simulink model "Simple_TDMA_test"  (Simulink 9.0)
settings: Solver=VariableStepAuto  StartTime=0.0  StopTime=1.0000e-04  RelTol=1e-3  EnableMultiTasking=on
undefined symbols (not defined in the file or in its folder): paramRFSatLink
libraries: commrflib2 x6, dspsigops x3, commrfcorlib x2, commrandsrc3 x2, dspsolvers x2, simulink x2, commfilt2 x2, commdigbbndam3 x2, commsink2 x1, commsync2 x1, commblksprivate x1
settings Model: SuppressorTable=22 serialization::archive 11 0 6 0 0 0 0 0  Creator=15337  LastModifiedBy=changgang
settings DataIOCC: LimitDataPoints=on  SaveFormat=Dataset
settings DebuggingCC: UnderspecifiedInitializationDetection=Simplified  MergeDetectMultiDrivingBlocksExec=error  AllowSymbolicDim=off
settings HardwareCC: ProdBitPerPointer=64  ProdBitPerSizeT=64  ProdBitPerPtrDiffT=64  ProdLargestAtomicFloat=Float  ProdIntDivRoundTo=Zero  ProdEndianess=LittleEndian  ProdWordSize=64  ProdHWDeviceType=Intel->x86-64 (Windows64)

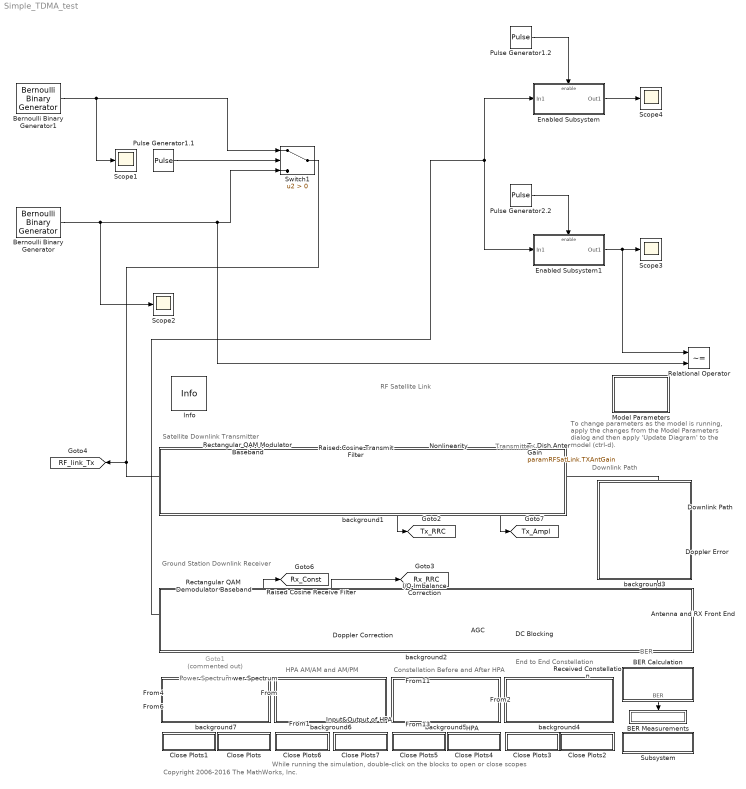
== system Simple_TDMA_test ==
  note: HPA AM/AM and AM/PM
  note: While running the simulation, double-click on the blocks to open or close scopes
  note: BER
  note: Power Spectrum
  note: Downlink Path
  note: RF Satellite Link
  note: Constellation Before and
      | After HPA
  note: End to End Constellation
  note: Ground Station Downlink Receiver
  note: Transmitter
  note: Satellite Downlink Transmitter
  note: Copyright 2006-2016 The MathWorks, Inc.
  note: To change parameters as the model is running, apply the changes from the Model Parameters dialog and then apply 'Update Diagram' to the model (ctrl-d).
  AGC : commrfcorlib/AGC  LegacyMode=off  DetectorMethod=Rectifier  LoopMethod=Linear  UpdatePeriod=100  StepSize=0.1  AdaptationStepSize=0.01  DesiredOutputPower=1  AveragingLength=256  MaximumGain=30  MaxPowerGain=400  GainOutputPort=off  InputPowerOutputPort=off  SimulateUsing=Code generation
      settings: SourceProductName=Communications System Toolbox
  Antenna and RX Front End : Subsystem
      mask Display: disp('Antenna and\nRX Front End')
  BER Calculation : Subsystem
      mask Display: disp('Display Complete\nBit Error Rate\nInformation');
  BER Measurements : Display
      settings: Format=short_e
  Bernoulli Binary Generator : commrandsrc3/Bernoulli Binary Generator  ProbabilityOfZero=0.5  SeedSource=Parameter  Seed=37  SampleTime=paramRFSatLink.sourceSampleTime  SamplesPerFrame=paramRFSatLink.sourceSamplesPerSymbol  OutputDataType=double  SimulateUsing=Interpreted execution
  Bernoulli Binary Generator1 : commrandsrc3/Bernoulli Binary Generator  ProbabilityOfZero=0.5  SeedSource=Parameter  Seed=37  SampleTime=paramRFSatLink.sourceSampleTime  SamplesPerFrame=paramRFSatLink.sourceSamplesPerSymbol  OutputDataType=double  SimulateUsing=Interpreted execution
  Close Plots : Subsystem
      settings: OpenFcn=|
      | sdspfscope2([],[],[],'ScopeUpdate',[bdroot '/Power Spectrum/Tx and Rx Spectrum'],'CloseFig');
      | set_param([bdroot '/Power Spectrum/Tx and Rx Spectrum'],'OpenScopeAtSimStart','off');
      mask Display: disp('Close Scopes');
  Close Plots1 : Subsystem
      settings: OpenFcn=|
      | sdspfscope2([],[],[],'ScopeUpdate',[bdroot '/Power Spectrum/Tx and Rx Spectrum'],'OpenFig');
      | set_param([bdroot '/Power Spectrum/Tx and Rx Spectrum'],'OpenScopeAtSimStart','on');
      mask Display: disp('Open Scopes');
  Close Plots2 : Subsystem
      settings: OpenFcn=|
      | sdspfscope2([],[],[],'ScopeUpdate',[bdroot '/Received Constellation'],'CloseFig');
      |    set_param([bdroot '/Received Constellation'],'OpenScopeAtSimStart','off');
      mask Display: disp('Close Scopes');
  Close Plots3 : Subsystem
      settings: OpenFcn=|
      | sdspfscope2([],[],[],'ScopeUpdate',[bdroot '/Received Constellation'],'OpenFig');
      |     set_param([bdroot '/Received Constellation'],'OpenScopeAtSimStart','on');
      mask Display: disp('Open Scopes');
  Close Plots4 : Subsystem
      settings: OpenFcn=|
      | sdspfscope2([],[],[],'ScopeUpdate',[bdroot '/HPA/Transmit RRC filtered signal'],'CloseFig');
      |   set_param([bdroot '/HPA/Transmit RRC filtered signal'],'OpenScopeAtSimStart','off');
      |     sdspfscope2([],[],[],'ScopeUpdate',[bdroot '/HPA/RRC signal after HPA'],'CloseFig');
      |   set_param([bdroot '/HPA/RRC signal after HPA'],'OpenScopeAtSimStart','off');
      mask Display: disp('Close Scopes');
  Close Plots5 : Subsystem
      settings: OpenFcn=|
      | sdspfscope2([],[],[],'ScopeUpdate',[bdroot '/HPA/Transmit RRC filtered signal'],'OpenFig');
      | set_param([bdroot '/HPA/Transmit RRC filtered signal'],'OpenScopeAtSimStart','on');
      |   sdspfscope2([],[],[],'ScopeUpdate',[bdroot '/HPA/RRC signal after HPA'],'OpenFig');
      | set_param([bdroot '/HPA/RRC signal after HPA'],'OpenScopeAtSimStart','on');
      mask Display: disp('Open Scopes');
  Close Plots6 : Subsystem
      settings: OpenFcn=|
      | sdspfscope2([],[],[],'ScopeUpdate',[bdroot '/Input&Output of HPA/HPA AM to AM'],'OpenFig');
      | set_param([bdroot '/Input&Output of HPA/HPA AM to AM'],'OpenScopeAtSimStart','on');
      | sdspfscope2([],[],[],'ScopeUpdate',[bdroot '/Input&Output of HPA/HPA AM to PM'],'OpenFig');
      | set_param([bdroot '/Input&Output of HPA/HPA AM to PM'],'OpenScopeAtSimStart','on');
      mask Display: disp('Open Scopes');
  Close Plots7 : Subsystem
      settings: OpenFcn=|
      | sdspfscope2([],[],[],'ScopeUpdate',[bdroot '/Input&Output of HPA/HPA AM to AM'],'CloseFig');
      | set_param([bdroot '/Input&Output of HPA/HPA AM to AM'],'OpenScopeAtSimStart','off');
      | sdspfscope2([],[],[],'ScopeUpdate',[bdroot '/Input&Output of HPA/HPA AM to PM'],'CloseFig');
      | set_param([bdroot '/Input&Output of HPA/HPA AM to PM'],'OpenScopeAtSimStart','off');
      mask Display: disp('Close Scopes');
  DC Blocking : Subsystem
      mask Display: disp('DC Blocking')
  Doppler Correction : Subsystem
      mask Display: disp('Doppler\nCorrection')
  Doppler Error : commrflib2/Phase// Frequency Offset  phaseOffset=0  freqPort=off  freqOffset=paramRFSatLink.DoppOffset
      settings: SourceProductName=Communications System Toolbox
  Downlink Path : commrflib2/Free Space Path Loss  mode=Distance and Frequency  dB=180  d=paramRFSatLink.Altitude  fc=paramRFSatLink.Frequency
      settings: SourceProductName=Communications System Toolbox  SourceProductBaseCode=CM
  Enabled Subsystem : Subsystem  TreatAsAtomicUnit=on
  Enabled Subsystem1 : Subsystem  TreatAsAtomicUnit=on
  Goto1 : Goto  Commented=on  GotoTag=RF_link_Rx  TagVisibility=global
  HPA : Subsystem  TreatAsAtomicUnit=on
      mask Display: disp('HPA\nConstellation')
  I/Q Imbalance Correction : Subsystem
      mask Display: disp('I/Q Imbalance\nCorrection')
  Info : commblksprivate/Info  SystemSampleTime=-1
      settings: SourceProductName=Communications System Toolbox  SourceProductBaseCode=CM
  Input&Output of HPA : Subsystem
      mask Display: disp('Input/Output\nof HPA')
  Model Parameters : Subsystem  mask(Model Parameters){altitude=35600, frequency=4000, antDiam=[.4 .4], selTemp=20 (very low noise level), selLvlBO=30 dB  (negligible nonlinearity), selDoppler=0 Hz, selNoPh=Negligible (-100 dBc/Hz @ 100 Hz), selImbal=None, selPreDistortion=off, selDcOffset=off, selCorrIQ=off, selCorrDoppler=off}
      mask prompts: altitude "Satellite altitude (km):"; frequency "Frequency (MHz):"; antDiam "Transmit and receive antenna diameters (m):"; selTemp "Noise temperature (K):"; selLvlBO "HPA backoff level:"; selDoppler "Doppler error:"; selNoPh "Phase noise:"; selImbal "I/Q imbalance and DC offset:"; selPreDistortion "Digital predistortion"; selDcOffset "DC offset correction"; selCorrIQ "I/Q imbalance correction"; selCorrDoppler "Doppler correction"
      mask help:
      | Select the scenarios from the mask to change the link parameters. Each of the mask parameters sets the parameters in the corresponding RF impairment or corresponding correction block(s).
      |
      | To make changes as the model is running, apply the changes from this dialog and then apply Update Diagram to the model (crtl-d).
      mask init:
      | commrfsatlink_mask(selLvlBO,selTemp, ...
      |     selDoppler, selImbal, selNoPh, ...
      |     selDcOffset, selCorrDoppler, selCorrIQ, altitude, ...
      |     frequency, antDiam,8,6,selPreDistortion);
      mask Help: helpview(commdhelp);
      mask TypeOptions selTemp: 0 (no noise) | 20 (very low noise level) | 290 (typical noise level) | 500 (high noise level)
      mask TypeOptions selLvlBO: 30 dB  (negligible nonlinearity) | 7 dB  (moderate nonlinearity) | 1 dB  (severe nonlinearity)
      mask TypeOptions selDoppler: 0 Hz | 3 Hz
      mask TypeOptions selNoPh: Negligible (-100 dBc/Hz @ 100 Hz) | Low  (-55 dBc/Hz @ 100 Hz) | High  (-48 dBc/Hz @ 100 Hz)
      mask TypeOptions selImbal: None | Amplitude imbalance (3 dB) | Phase imbalance (20 deg) | In-phase DC offset (2e-6) | Quadrature DC offset (1e-5)
      mask Display: disp('Model\nParameters');
  Nonlinearity : Subsystem
      mask Display: disp('HPA\n Nonlinearity\n with Optional\n Digital\nPredistortion')
  Power Spectrum : Subsystem  TreatAsAtomicUnit=on
      mask Display: disp('Power\nSpectrum')
  Pulse Generator1.1 : DiscretePulseGenerator  PulseType=Time based  Period=5.0000e-06  PulseWidth=50
  "Pulse Generator1.2 " : DiscretePulseGenerator  PulseType=Time based  Period=1.0000e-05  PulseWidth=50
  Pulse Generator2.2 : DiscretePulseGenerator  PulseType=Time based  Period=1.0000e-05  PulseWidth=50  PhaseDelay=0.05
  Raised Cosine Receive Filter : commfilt2/Raised Cosine Receive Filter  filtType=Square root  R=0.3  filtSpan=paramRFSatLink.FilterSpan  N=paramRFSatLink.SamplesPerSymbol  downFactor=paramRFSatLink.SamplesPerSymbol  downOffset=0  filterGain=1/sqrt(paramRFSatLink.SamplesPerSymbol)  InputProcessing=Columns as channels (frame based)  RateOptions=Enforce single-rate processing  framing=Mute  checkCoeff=off  variableName=rcRxFilt  currentFiltSpan=2*((2*(3))/2)  D=(2*(3))/2  inputOffset=0  sampMode=Mute  saveAsFlag=0  rateMode=Downsampling  checkGain=Normalized  launchFVT=off  roundingMode=Floor  overflowMode=off  coeffDataTypeStr=Inherit: Same word length as input  coeffMin=[]  coeffMax=[]  coeffLastDataTypeStr=Inherit: Same word length as input  accumDataTypeStr=Inherit: Same as product output  accumLastDataTypeStr=Inherit: Same as product output  outputDataTypeStr=Inherit: Same as accumulator  outputMin=[]  outputMax=[]  outputLastDataTypeStr=Inherit: Same as accumulator
  Raised Cosine Transmit Filter : commfilt2/Raised Cosine Transmit Filter  filtType=Square root  R=0.3  filtSpan=paramRFSatLink.FilterSpan  N=paramRFSatLink.SamplesPerSymbol  filterGain=sqrt(paramRFSatLink.SamplesPerSymbol)  InputProcessing=Columns as channels (frame based)  RateOptions=Enforce single-rate processing  framing=Mute  checkCoeff=off  variableName=rcTxFilt  checkGain=Normalized  sampMode=Mute  saveAsFlag=0  currentFiltSpan=2*((2*(3))/2)  D=(2*(3))/2  launchFVT=off  roundingMode=Floor  overflowMode=off  coeffDataTypeStr=Inherit: Same word length as input  coeffMin=[]  coeffMax=[]  coeffLastDataTypeStr=Inherit: Same word length as input  outputDataTypeStr=Inherit: Same as accumulator  outputMin=[]  outputMax=[]  outputLastDataTypeStr=Inherit: Same as accumulator
  Received Constellation : ConstellationDiagram  Tag=ScatterPlot
  Rectangular QAM Demodulator Baseband : commdigbbndam3/Rectangular QAM Demodulator Baseband  M=16  OutType=Bit  DecType=Hard decision  VarSource=Dialog  Variance=1  Dec=Gray  Mapping=[0:15]  PowType=Average Power  MinDist=2  AvgPow=1  PeakPow=1  Ph=0  outDtype1=boolean  outDtype2=double  derotateFactorWordLen=16  derotateFactorDataTypeStr=Inherit: Same word length as input  derotateFactorLastDataTypeStr=Inherit: Same word length as input  denormFactorWordLen=16  denormFactorDataTypeStr=Inherit: Same word length as input  denormFactorLastDataTypeStr=Inherit: Same word length as input  prodOutWordLen=32  prodOutOverflowMode=Wrap  prodOutRoundingMode=Floor  prodOutOvFlMode=off  prodOutOvFlModeLastStrValue=off  sumWordLen=32
  Rectangular QAM Modulator Baseband : commdigbbndam3/Rectangular QAM Modulator Baseband  M=16  InType=Bit  Enc=Gray  Mapping=[0:15]  PowType=Average Power  MinDist=2  AvgPow=1  PeakPow=1  Ph=0  outDtype=double  outWordLen=16  outUDDataType=sfix(16)  outFracLenMode=Best precision  outFracLen=15  outDataTypeStr=double  outLastDataTypeStr=double
  Relational Operator : RelationalOperator  Operator=~=  OutDataTypeStr=boolean  RndMeth=Nearest
  Scope{1..4} (4 alike) : Scope
  Subsystem : Subsystem
      settings: OpenFcn=|
      | % Set value to reset BER
      | warning('off', 'Simulink:Engine:NonTunableVarChanged');
      | paramRFSatLink.resetBER = 1;
      | set_param(bdroot, 'SimulationCommand', 'update');
      | pause(0.1)
      | 
      | % Set value so that BER is not continually reset
      | paramRFSatLink.resetBER = 0;
      | set_param(bdroot, 'SimulationCommand', 'update');
      | warning('on', 'Simulink:Engine:NonTunableVarChanged');
      mask Display: disp('Double-click to\nreset BER')
  Switch1 : Switch  Criteria=u2 > Threshold
  Tx Dish Antenna Gain : Gain  Gain=paramRFSatLink.TXAntGain  SaturateOnIntegerOverflow=on  OutDataTypeStr=Inherit: Same as input  ParamDataTypeStr=Inherit: Same as input
  background1 : Subsystem
      mask Display: disp('')
  background2 : Subsystem
      mask Display: disp('')
  background3 : Subsystem
      mask Display: disp('')
  background4 : Subsystem
      mask Display: disp('')
  background5 : Subsystem
      mask Display: disp('')
  background6 : Subsystem
      mask Display: disp('')
  background7 : Subsystem
      mask Display: disp('')
  tag scope: RF_link_Tx=global, Rx_Const=global, Rx_RRC=global, Tx_Ampl=global, Tx_RRC=global
  wires:
  Pulse Generator1.1/1 -> Switch1/2
  "Pulse Generator1.2 "/1 -> Enabled Subsystem/Enable
  Pulse Generator2.2/1 -> Enabled Subsystem1/Enable
  Bernoulli Binary Generator/1 -> Relational Operator/2, Switch1/3, Scope2/1
  Rectangular QAM Demodulator Baseband/1 -> Enabled Subsystem1/1(In1), Enabled Subsystem/1(In1), Goto1/1
  Enabled Subsystem/1(Out1) -> Scope4/1
  Enabled Subsystem1/1(Out1) -> Relational Operator/1, Scope3/1
  Antenna and RX Front End/1(Out1) -> DC Blocking/1(In1)
  [Tx_Ampl] -> HPA/2(In3)
  BER Calculation/1(BER) -> BER Measurements/1
  [HPA_Out] -> Input&Output of HPA/2(In2)
  [Rx_Const] -> Received Constellation/1
  Doppler Correction/1(Out1) -> [Rx_RRC], Raised Cosine Receive Filter/1
  Downlink Path/1 -> Doppler Error/1
  Raised Cosine Receive Filter/1 -> [Rx_Const], Rectangular QAM Demodulator Baseband/1
  Tx Dish Antenna Gain/1 -> Downlink Path/1
  Doppler Error/1 -> Antenna and RX Front End/1(In1)
  DC Blocking/1(Out1) -> AGC/1
  Switch1/1 -> Rectangular QAM Modulator Baseband/1, [RF_link_Tx]
  [Tx_RRC] -> HPA/1(In2)
  I/Q Imbalance Correction/1(Out1) -> Doppler Correction/1(In1)
  AGC/1 -> I/Q Imbalance Correction/1(In1)
  [HPA_In] -> Input&Output of HPA/1(In1)
  [Rx_RRC] -> Power Spectrum/2(In2)
  Nonlinearity/1(Out2) -> [Tx_Ampl], Tx Dish Antenna Gain/1
  [Tx_RRC] -> Power Spectrum/1(In1)
  Raised Cosine Transmit Filter/1 -> [Tx_RRC], Nonlinearity/1(In)
  Bernoulli Binary Generator1/1 -> Switch1/1, Scope1/1
  Rectangular QAM Modulator Baseband/1 -> Raised Cosine Transmit Filter/1

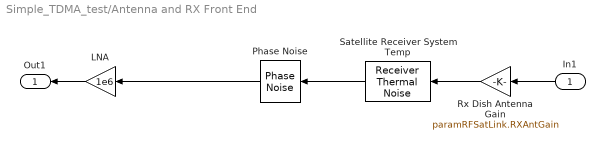
== system Simple_TDMA_test/Antenna and RX Front End ==
  In1 : Inport
  LNA : Gain  Gain=1e6
  Phase Noise : commrflib2/Phase Noise  PhNs=paramRFSatLink.PhaseNoise  Fo=100  Fs=2e5  seed=2137
      settings: SourceProductName=Communications System Toolbox  SourceProductBaseCode=CM
  Rx Dish Antenna Gain : Gain  Gain=paramRFSatLink.RXAntGain  SaturateOnIntegerOverflow=on  OutDataTypeStr=Inherit: Same as input  ParamDataTypeStr=Inherit: Same as input
  Satellite Receiver System Temp : commrflib2/Receiver Thermal Noise  method=Noise temperature  ntemp=paramRFSatLink.RXTemp  nfigure=20  nfactor=2  add290KAntennaNoise=off  seed=67987
      settings: SourceProductName=Communications System Toolbox  SourceProductBaseCode=CM
  Out1 : Outport
  wires:
  LNA/1 -> Out1/1
  Satellite Receiver System Temp/1 -> Phase Noise/1
  In1/1 -> Rx Dish Antenna Gain/1
  Phase Noise/1 -> LNA/1
  Rx Dish Antenna Gain/1 -> Satellite Receiver System Temp/1

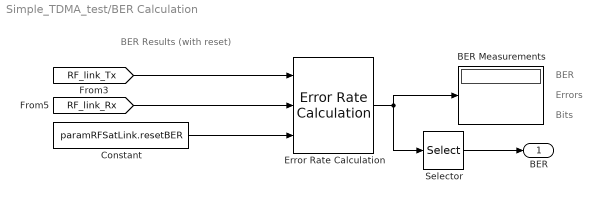
== system Simple_TDMA_test/BER Calculation ==
  note: BER
  note: Errors
  note: Bits
  note: BER Results (with reset)
  BER Measurements : Display
  Constant : Constant  Value=paramRFSatLink.resetBER  SampleTime=paramRFSatLink.sourceSampleTime * paramRFSatLink.sourceSamplesPerSymbol
  Error Rate Calculation : commsink2/Error Rate Calculation  N=24  st_delay=0  cp_mode=Entire frame  subframe=[]  PMode=Port  WsName=ErrorVec  RsMode2=on  stop=off  numErr=200  maxBits=1e6
  Selector : Selector  InputPortWidth=3  IndexOptions=Index vector (dialog)  Indices=[1]  OutputSizes=1
  BER : Outport
  wires:
  [RF_link_Rx] -> Error Rate Calculation/2
  Error Rate Calculation/1 -> Selector/1, BER Measurements/1
  Constant/1 -> Error Rate Calculation/3
  Selector/1 -> BER/1
  [RF_link_Tx] -> Error Rate Calculation/1

== system Simple_TDMA_test/Close Plots ==

== system Simple_TDMA_test/Close Plots1 ==

== system Simple_TDMA_test/Close Plots2 ==

== system Simple_TDMA_test/Close Plots3 ==

== system Simple_TDMA_test/Close Plots4 ==

== system Simple_TDMA_test/Close Plots5 ==

== system Simple_TDMA_test/Close Plots6 ==

== system Simple_TDMA_test/Close Plots7 ==

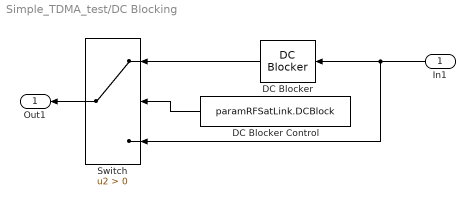
== system Simple_TDMA_test/DC Blocking ==
  In1 : Inport
  DC Blocker : dspsigops/DC Blocker  Algorithm=IIR  NormalizedBandwidth=0.0005  Length=8  Order=6  SimulateUsing=Code generation
      settings: SourceProductName=DSP System Toolbox  SourceProductBaseCode=DS
  DC Blocker Control : Constant  Value=paramRFSatLink.DCBlock  SampleTime=paramRFSatLink.sourceSampleTime * paramRFSatLink.sourceSamplesPerSymbol
  Switch : Switch  Criteria=u2 > Threshold
  Out1 : Outport
  wires:
  In1/1 -> Switch/3, DC Blocker/1
  DC Blocker Control/1 -> Switch/2
  Switch/1 -> Out1/1
  DC Blocker/1 -> Switch/1

== system Simple_TDMA_test/Doppler Correction ==
  In1 : Inport
  Carrier Synchronizer : commsync2/Carrier Synchronizer  Modulation=QAM  ModulationPhaseOffset=Auto  CustomPhaseOffset=0  SamplesPerSymbol=paramRFSatLink.SamplesPerSymbol  DampingFactor=0.707  NormalizedLoopBandwidth=0.01  EstimatedPhaseErrorOutputPort=off  SimulateUsing=Code generation
      settings: SourceProductName=Communications System Toolbox
  Doppler Correction : Constant  Value=paramRFSatLink.CarrierSync  SampleTime=paramRFSatLink.sourceSampleTime * paramRFSatLink.sourceSamplesPerSymbol
  Switch : Switch  Criteria=u2 > Threshold
  Out1 : Outport
  wires:
  Doppler Correction/1 -> Switch/2
  Carrier Synchronizer/1 -> Switch/1
  Switch/1 -> Out1/1
  In1/1 -> Carrier Synchronizer/1, Switch/3

== system Simple_TDMA_test/Enabled Subsystem ==
  In1 : Inport
  Enable : EnablePort
  Out1 : Outport
  wires:
  In1/1 -> Out1/1

== system Simple_TDMA_test/Enabled Subsystem1 ==
  In1 : Inport
  Enable : EnablePort
  Out1 : Outport
  wires:
  In1/1 -> Out1/1

== system Simple_TDMA_test/HPA ==
  In2 : Inport
  In3 : Inport  Port=2
  RRC signal after HPA : ConstellationDiagram
  Transmit RRC filtered signal : ConstellationDiagram
  wires:
  In2/1 -> Transmit RRC filtered signal/1
  In3/1 -> RRC signal after HPA/1

== system Simple_TDMA_test/I/Q Imbalance Correction ==
  In1 : Inport
  I/Q Imbalance Compensator : commrfcorlib/I//Q Imbalance Compensator  CoefficientSource=Estimated from input signal  InitialCoefficient=0 + 0j  StepSizeSource=Property  StepSize=0.00001  AdaptInputPort=off  CoefficientOutputPort=off  SimulateUsing=Code generation
      settings: SourceProductName=Communications System Toolbox  SourceProductBaseCode=CM
  I/Q Imbalance Correction : Constant  Value=paramRFSatLink.IQComp  SampleTime=paramRFSatLink.sourceSampleTime * paramRFSatLink.sourceSamplesPerSymbol
  Switch : Switch  Criteria=u2 > Threshold
  Out1 : Outport
  wires:
  I/Q Imbalance Correction/1 -> Switch/2
  I/Q Imbalance Compensator/1 -> Switch/1
  Switch/1 -> Out1/1
  In1/1 -> I/Q Imbalance Compensator/1, Switch/3

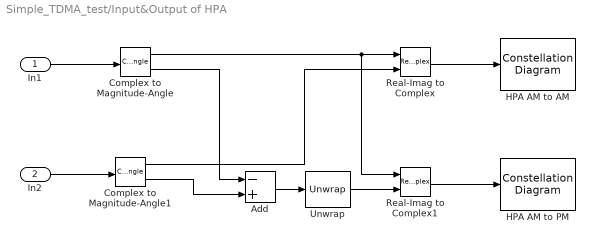
== system Simple_TDMA_test/Input&Output of HPA ==
  In1 : Inport
  In2 : Inport  Port=2
  Add : Sum  Inputs=-+
  Complex to Magnitude-Angle : ComplexToMagnitudeAngle
  Complex to Magnitude-Angle1 : ComplexToMagnitudeAngle
  HPA AM to AM : ConstellationDiagram  Tag=ScatterPlot
  HPA AM to PM : ConstellationDiagram  Tag=ScatterPlot
  Real-Imag to Complex : RealImagToComplex
  Real-Imag to Complex1 : RealImagToComplex
  Unwrap : dspsigops/Unwrap  tol=pi  InputProcessing=Columns as channels (frame based)  running=on
  wires:
  Real-Imag to Complex/1 -> HPA AM to AM/1
  Complex to Magnitude-Angle1/1 -> Real-Imag to Complex/2
  Add/1 -> Unwrap/1
  In1/1 -> Complex to Magnitude-Angle/1
  In2/1 -> Complex to Magnitude-Angle1/1
  Real-Imag to Complex1/1 -> HPA AM to PM/1
  Unwrap/1 -> Real-Imag to Complex1/2
  Complex to Magnitude-Angle1/2 -> Add/2
  Complex to Magnitude-Angle/1 -> Real-Imag to Complex1/1, Real-Imag to Complex/1
  Complex to Magnitude-Angle/2 -> Add/1

== system Simple_TDMA_test/Model Parameters ==

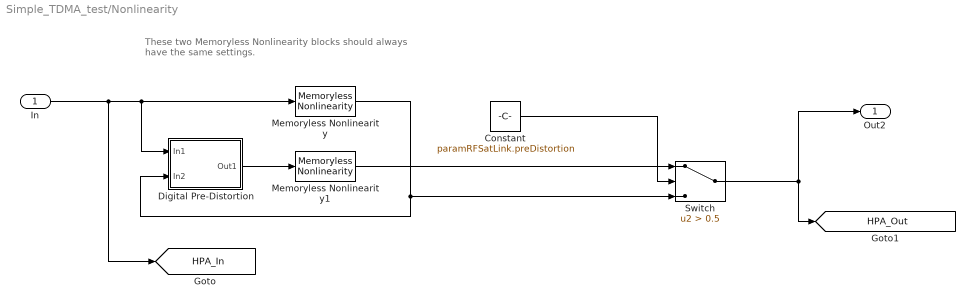
== system Simple_TDMA_test/Nonlinearity ==
  note: These two Memoryless Nonlinearity blocks should always
      | have the same settings.
  In : Inport
  Constant : Constant  Value=paramRFSatLink.preDistortion  VectorParams1D=off  SampleTime=paramRFSatLink.sourceSampleTime * paramRFSatLink.sourceSamplesPerSymbol
  Digital Pre-Distortion : Subsystem
      mask Display: disp('Digital\nPredistortion')
  Memoryless Nonlinearity : commrflib2/Memoryless Nonlinearity  model_select=Saleh model  linGaindB=0  GindB=paramRFSatLink.GindB  iip3=30  am2pm=10  LPwrLimAMPM=10  UPwrLimAMPM=inf  amam=[2.1587 1.1517]  ampm=[4.0330 9.1040]  x=[8.1081 1.5413 6.5202 -0.0718]  y=[4.6645 2.0965 10.88 -0.003]  p=0.5  GoutdB=paramRFSatLink.GoutdB  vsat=1
      settings: SourceProductName=Communications System Toolbox  SourceProductBaseCode=CM
  Memoryless Nonlinearity1 : commrflib2/Memoryless Nonlinearity  model_select=Saleh model  linGaindB=0  GindB=paramRFSatLink.GindB  iip3=30  am2pm=10  LPwrLimAMPM=10  UPwrLimAMPM=inf  amam=[2.1587 1.1517]  ampm=[4.0330 9.1040]  x=[8.1081 1.5413 6.5202 -0.0718]  y=[4.6645 2.0965 10.88 -0.003]  p=0.5  GoutdB=paramRFSatLink.GoutdB  vsat=1
      settings: SourceProductName=Communications System Toolbox  SourceProductBaseCode=CM
  Switch : Switch  Criteria=u2 > Threshold  Threshold=0.5  ZeroCross=off
  Out2 : Outport
  tag scope: HPA_In=global, HPA_Out=global
  wires:
  Digital Pre-Distortion/1(Out1) -> Memoryless Nonlinearity1/1
  Memoryless Nonlinearity/1 -> Switch/3, Digital Pre-Distortion/2(In2)
  Switch/1 -> Out2/1, [HPA_Out]
  In/1 -> [HPA_In], Memoryless Nonlinearity/1, Digital Pre-Distortion/1(In1)
  Constant/1 -> Switch/2
  Memoryless Nonlinearity1/1 -> Switch/1

== system Simple_TDMA_test/Power Spectrum ==
  In1 : Inport
  In2 : Inport  Port=2
  Matrix Concatenation : Concatenate  Mode=Multidimensional array  ConcatenateDimension=2
  Tx and Rx Spectrum : SpectrumAnalyzer
  wires:
  In1/1 -> Matrix Concatenation/1
  In2/1 -> Matrix Concatenation/2
  Matrix Concatenation/1 -> Tx and Rx Spectrum/1

== system Simple_TDMA_test/Subsystem ==

== system Simple_TDMA_test/background1 ==

== system Simple_TDMA_test/background2 ==

== system Simple_TDMA_test/background3 ==

== system Simple_TDMA_test/background4 ==

== system Simple_TDMA_test/background5 ==

== system Simple_TDMA_test/background6 ==

== system Simple_TDMA_test/background7 ==

== system Simple_TDMA_test/Nonlinearity/Digital Pre-Distortion ==
  In1 : Inport
  In2 : Inport  Port=2
  Distortion compensation : Subsystem
  Parameter Estimation : Subsystem
  Out1 : Outport
  wires:
  In2/1 -> Parameter Estimation/2(DUT Output)
  Distortion compensation/1(Pre-distorted Signal) -> Out1/1
  Parameter Estimation/2(d) -> Distortion compensation/2(d)
  Parameter Estimation/1(c) -> Distortion compensation/1(c)
  In1/1 -> Parameter Estimation/1(DUT Input), Distortion compensation/3(In)

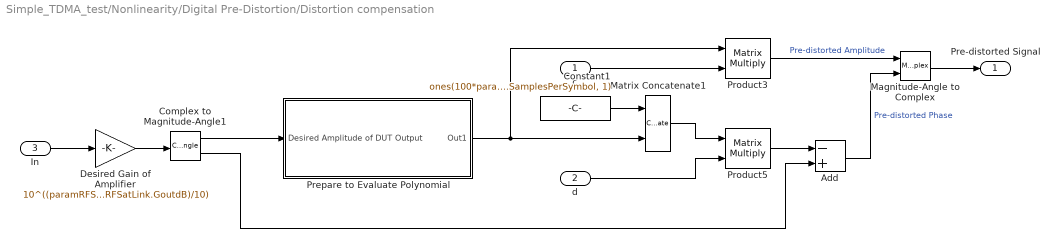
== system Simple_TDMA_test/Nonlinearity/Digital Pre-Distortion/Distortion compensation ==
  c : Inport
  d : Inport  Port=2
  In : Inport  Port=3
  Add : Sum  Inputs=-+
  Complex to Magnitude-Angle1 : ComplexToMagnitudeAngle
  Constant1 : Constant  Value=ones(100*paramRFSatLink.SamplesPerSymbol, 1)
  Desired Gain of Amplifier : Gain  Gain=10^((paramRFSatLink.GindB + paramRFSatLink.GoutdB)/10)
  Magnitude-Angle to Complex : MagnitudeAngleToComplex
  Matrix Concatenate1 : Concatenate  Mode=Multidimensional array  ConcatenateDimension=2
  Prepare to Evaluate Polynomial : Subsystem
  Product3 : Product  Multiplication=Matrix(*)  RndMeth=Zero
  Product5 : Product  Multiplication=Matrix(*)  RndMeth=Zero
  Pre-distorted Signal : Outport
  wires:
  Constant1/1 -> Matrix Concatenate1/1
  Prepare to Evaluate Polynomial/1(Out1) -> Product3/1, Matrix Concatenate1/2
  Matrix Concatenate1/1 -> Product5/1
  Complex to Magnitude-Angle1/1 -> Prepare to Evaluate Polynomial/1(Desired Amplitude of DUT Output)
  Complex to Magnitude-Angle1/2 -> Add/2
  Magnitude-Angle to Complex/1 -> Pre-distorted Signal/1
  In/1 -> Desired Gain of Amplifier/1
  d/1 -> Product5/2
  Product3/1 -> Magnitude-Angle to Complex/1  "Pre-distorted Amplitude"
  Product5/1 -> Add/1
  Add/1 -> Magnitude-Angle to Complex/2  "Pre-distorted Phase"
  c/1 -> Product3/2
  Desired Gain of Amplifier/1 -> Complex to Magnitude-Angle1/1

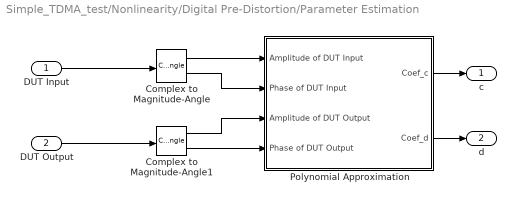
== system Simple_TDMA_test/Nonlinearity/Digital Pre-Distortion/Parameter Estimation ==
  DUT Input : Inport
  DUT Output : Inport  Port=2
  Complex to Magnitude-Angle : ComplexToMagnitudeAngle
  Complex to Magnitude-Angle1 : ComplexToMagnitudeAngle
  Polynomial Approximation : Subsystem
  c : Outport
  d : Outport  Port=2
  wires:
  Complex to Magnitude-Angle/1 -> Polynomial Approximation/1(Amplitude of DUT Input)
  Complex to Magnitude-Angle1/2 -> Polynomial Approximation/4(Phase of DUT Output)
  Polynomial Approximation/2(Coef_d) -> d/1
  Polynomial Approximation/1(Coef_c) -> c/1
  Complex to Magnitude-Angle/2 -> Polynomial Approximation/2(Phase of DUT Input)
  Complex to Magnitude-Angle1/1 -> Polynomial Approximation/3(Amplitude of DUT Output)
  DUT Output/1 -> Complex to Magnitude-Angle1/1
  DUT Input/1 -> Complex to Magnitude-Angle/1

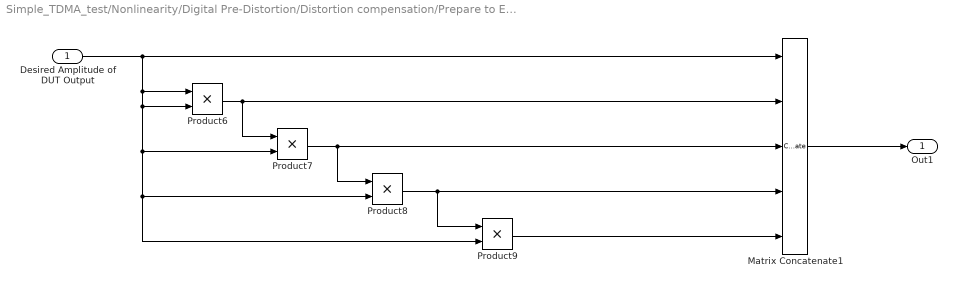
== system Simple_TDMA_test/Nonlinearity/Digital Pre-Distortion/Distortion compensation/Prepare to Evaluate Polynomial ==
  Desired Amplitude of DUT Output : Inport
  Matrix Concatenate1 : Concatenate  NumInputs=5  Mode=Multidimensional array  ConcatenateDimension=2
  Product{6..9} (4 alike) : Product  RndMeth=Zero
  Out1 : Outport
  wires:
  Matrix Concatenate1/1 -> Out1/1
  Product9/1 -> Matrix Concatenate1/5
  Product8/1 -> Matrix Concatenate1/4, Product9/1
  Product6/1 -> Matrix Concatenate1/2, Product7/1
  Product7/1 -> Matrix Concatenate1/3, Product8/1
  Desired Amplitude of DUT Output/1 -> Matrix Concatenate1/1, Product6/1, Product6/2, Product7/2, Product8/2, Product9/2

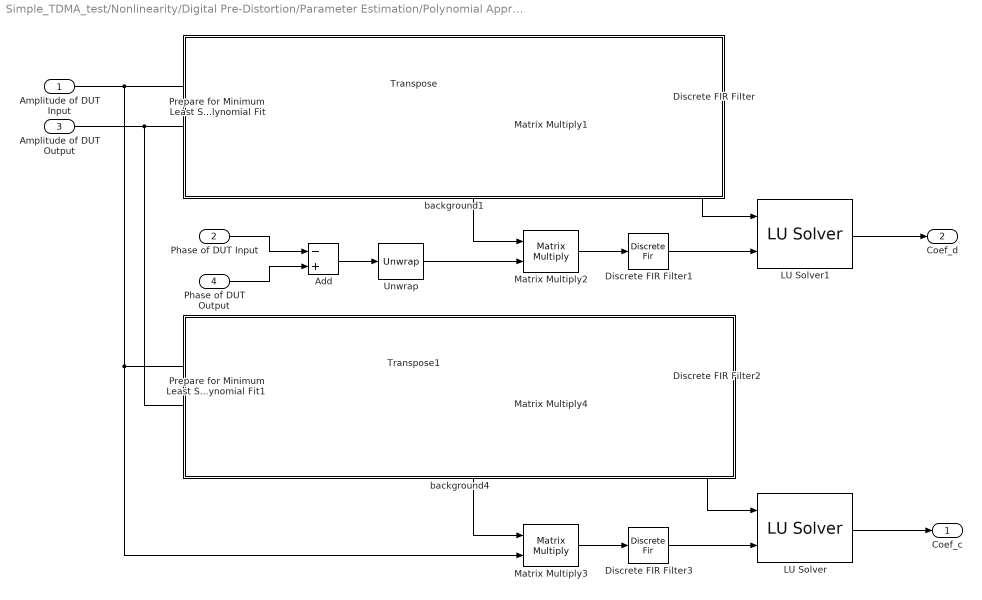
== system Simple_TDMA_test/Nonlinearity/Digital Pre-Distortion/Parameter Estimation/Polynomial Approximation ==
  Amplitude of DUT Input : Inport
  Phase of DUT Input : Inport  Port=2
  Amplitude of DUT Output : Inport  Port=3
  Phase of DUT Output : Inport  Port=4
  Add : Sum  Inputs=-+
  Discrete FIR Filter{,1..3} (4 alike) : DiscreteFir  Coefficients=ones(1,50)  AccumDataTypeStr=Inherit: Same as product output
  LU Solver : dspsolvers/LU Solver
      settings: SourceProductName=DSP System Toolbox  SourceProductBaseCode=DS
  LU Solver1 : dspsolvers/LU Solver
      settings: SourceProductName=DSP System Toolbox  SourceProductBaseCode=DS
  Matrix Multiply{1..4} (4 alike) : Product  Multiplication=Matrix(*)
  Prepare for Minimum Least Square Error Polynomial Fit : Subsystem
  Prepare for Minimum Least Square Error Polynomial Fit1 : Subsystem
  Transpose : Math  Operator=transpose  SaturateOnIntegerOverflow=on
  Transpose1 : Math  Operator=transpose  SaturateOnIntegerOverflow=on
  Unwrap : dspsigops/Unwrap  tol=pi  InputProcessing=Columns as channels (frame based)  running=off
  background1 : Subsystem
      mask Display: disp('')
  background4 : Subsystem
      mask Display: disp('')
  Coef_c : Outport
  Coef_d : Outport  Port=2
  wires:
  Transpose/1 -> Matrix Multiply2/1, Matrix Multiply1/1
  LU Solver/1 -> Coef_c/1
  LU Solver1/1 -> Coef_d/1
  Phase of DUT Output/1 -> Add/2
  Discrete FIR Filter3/1 -> LU Solver/2
  Discrete FIR Filter/1 -> LU Solver1/1
  Discrete FIR Filter1/1 -> LU Solver1/2
  Amplitude of DUT Output/1 -> Prepare for Minimum Least Square Error Polynomial Fit/2(In2), Prepare for Minimum Least Square Error Polynomial Fit1/2(In2)
  Matrix Multiply2/1 -> Discrete FIR Filter1/1
  Unwrap/1 -> Matrix Multiply2/2
  Prepare for Minimum Least Square Error Polynomial Fit/1(Out1) -> Transpose/1, Matrix Multiply1/2
  Matrix Multiply3/1 -> Discrete FIR Filter3/1
  Matrix Multiply1/1 -> Discrete FIR Filter/1
  Amplitude of DUT Input/1 -> Matrix Multiply3/2, Prepare for Minimum Least Square Error Polynomial Fit1/1(In1), Prepare for Minimum Least Square Error Polynomial Fit/1(In1)
  Add/1 -> Unwrap/1
  Phase of DUT Input/1 -> Add/1
  Prepare for Minimum Least Square Error Polynomial Fit1/1(Out1) -> Transpose1/1, Matrix Multiply4/2
  Matrix Multiply4/1 -> Discrete FIR Filter2/1
  Transpose1/1 -> Matrix Multiply4/1, Matrix Multiply3/1
  Discrete FIR Filter2/1 -> LU Solver/1

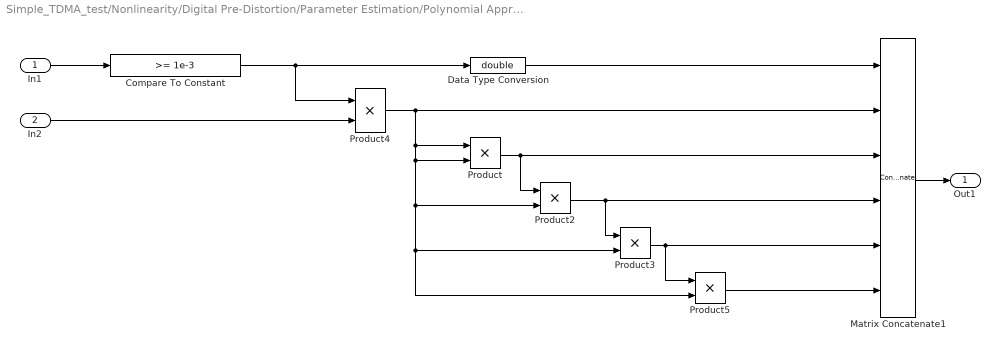
== system Simple_TDMA_test/Nonlinearity/Digital Pre-Distortion/Parameter Estimation/Polynomial Approximation/Prepare for Minimum Least Square Error Polynomial Fit ==
  In1 : Inport
  In2 : Inport  Port=2
  Compare To Constant : simulink/Logic and Bit Operations/Compare To Constant  relop=>=  const=1e-3  OutDataTypeStr=uint8  ZeroCross=off
  Data Type Conversion : DataTypeConversion  OutDataTypeStr=double
  Matrix Concatenate1 : Concatenate  NumInputs=6  Mode=Multidimensional array  ConcatenateDimension=2
  Product{,2..5} (5 alike) : Product  RndMeth=Zero
  Out1 : Outport
  wires:
  Data Type Conversion/1 -> Matrix Concatenate1/1
  In1/1 -> Compare To Constant/1
  Matrix Concatenate1/1 -> Out1/1
  Product5/1 -> Matrix Concatenate1/6
  Product4/1 -> Product/1, Product/2, Product2/2, Product3/2, Product5/2, Matrix Concatenate1/2
  Product/1 -> Matrix Concatenate1/3, Product2/1
  Product2/1 -> Matrix Concatenate1/4, Product3/1
  Product3/1 -> Matrix Concatenate1/5, Product5/1
  In2/1 -> Product4/2
  Compare To Constant/1 -> Data Type Conversion/1, Product4/1

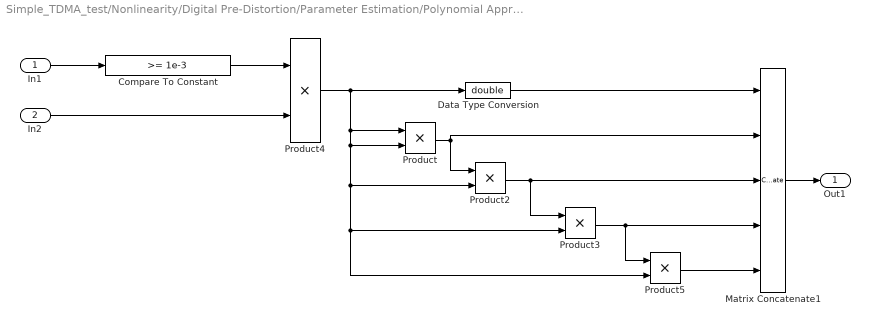
== system Simple_TDMA_test/Nonlinearity/Digital Pre-Distortion/Parameter Estimation/Polynomial Approximation/Prepare for Minimum Least Square Error Polynomial Fit1 ==
  In1 : Inport
  In2 : Inport  Port=2
  Compare To Constant : simulink/Logic and Bit Operations/Compare To Constant  relop=>=  const=1e-3  OutDataTypeStr=uint8  ZeroCross=off
  Data Type Conversion : DataTypeConversion  OutDataTypeStr=double
  Matrix Concatenate1 : Concatenate  NumInputs=5  Mode=Multidimensional array  ConcatenateDimension=2
  Product{,2..5} (5 alike) : Product  RndMeth=Zero
  Out1 : Outport
  wires:
  In1/1 -> Compare To Constant/1
  Matrix Concatenate1/1 -> Out1/1
  Product2/1 -> Product3/1, Matrix Concatenate1/3
  Product3/1 -> Product5/1, Matrix Concatenate1/4
  Product5/1 -> Matrix Concatenate1/5
  Product4/1 -> Product/1, Product/2, Product5/2, Product3/2, Product2/2, Data Type Conversion/1
  Product/1 -> Product2/1, Matrix Concatenate1/2
  In2/1 -> Product4/2
  Data Type Conversion/1 -> Matrix Concatenate1/1
  Compare To Constant/1 -> Product4/1

== system Simple_TDMA_test/Nonlinearity/Digital Pre-Distortion/Parameter Estimation/Polynomial Approximation/background1 ==

== system Simple_TDMA_test/Nonlinearity/Digital Pre-Distortion/Parameter Estimation/Polynomial Approximation/background4 ==
